simulink model "BT02"  (R2026b)
settings: Solver=ode45  StopTime=cfg.stop_s  MaxStep=cfg.max_step_s  RelTol=1e-10  AbsTol=1e-12
PostLoadFcn:
  | addpath(fileparts(get_param(bdroot,'FileName')));load_case('BT02');
InitFcn:
  | addpath(fileparts(get_param(bdroot,'FileName')));load_case('BT02');
values from neighbouring files (symbols this model uses):
  cfg = jsondecode(fileread(fullfile(root,'fixtures',[id '.json'])))    [load_case.m]
undefined symbols (not defined in the file or in its folder): capacity_Ah, pack_count, solar_gain
settings Model: Creator=markl  LastModifiedBy=markl
settings DataIOCC: SaveOutput=off

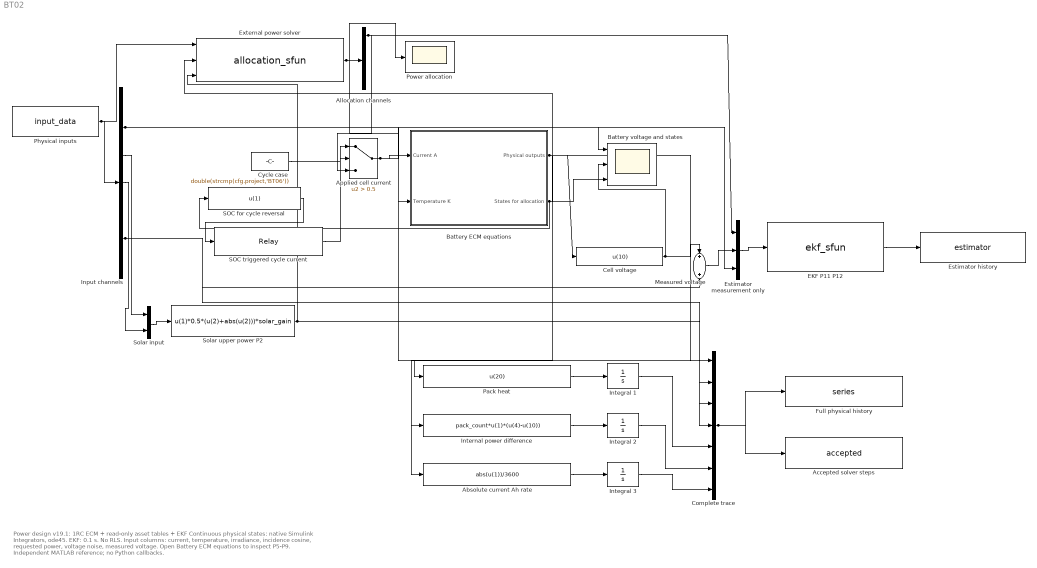
== system BT02 ==
  note: Power design v19.1: 1RC ECM + read-only asset tables + EKF
      | Continuous physical states: native Simulink Integrators, ode45. EKF: 0.1 s. No RLS.
      | Input columns: current, temperature, irradiance, incidence cosine, requested power, voltage noise, measured voltage.
      | Open Battery ECM equations to inspect P5-P9. Independent MATLAB reference; no Python callbacks.
  Absolute current Ah rate : Fcn  Expr=abs(u(1))/3600
  Accepted solver steps : ToWorkspace  VariableName=accepted  SaveFormat=Structure With Time  SampleTime=-1
  Allocation channels : Demux  Outputs=6
  Applied cell current : Switch  Criteria=u2 > Threshold  Threshold=0.5  SaturateOnIntegerOverflow=off  InputSameDT=off
  Battery ECM equations : Subsystem
  Battery voltage and states : Scope  NumInputPorts=3
  Cell voltage : Fcn  Expr=u(10)
  Complete trace : Mux  Inputs=7
  Cycle case : Constant  Value=double(strcmp(cfg.project,'BT06'))
  EKF P11 P12 : M-S-Function  FunctionName=ekf_sfun  Parameters=cfg
  Estimator history : ToWorkspace  VariableName=estimator  SaveFormat=Structure With Time  SampleTime=cfg.dt_s
  Estimator measurement only : Mux  Inputs=3
  External power solver : M-S-Function  FunctionName=allocation_sfun  Parameters=cfg
  Full physical history : ToWorkspace  VariableName=series  SaveFormat=Structure With Time  SampleTime=cfg.dt_s
  Input channels : Demux  Outputs=7
  Integral 1 : Integrator
  Integral 2 : Integrator
  Integral 3 : Integrator
  Internal power difference : Fcn  Expr=pack_count*u(1)*(u(4)-u(10))
  Measured voltage : Sum
  Pack heat : Fcn  Expr=u(20)
  Physical inputs : FromWorkspace  VariableName=input_data  SampleTime=cfg.dt_s  Interpolate=off  OutputAfterFinalValue=Holding final value
  Power allocation : Scope
  SOC for cycle reversal : Fcn  Expr=u(1)
  SOC triggered cycle current : Relay  OnSwitchValue=0.88  OffSwitchValue=0.1  OnOutputValue=0.2  OffOutputValue=-0.2
  Solar input : Mux  Inputs=2
  Solar upper power P2 : Fcn  Expr=u(1)*0.5*(u(2)+abs(u(2)))*solar_gain
  wires:
  Physical inputs/1 -> Input channels/1, External power solver/1
  Input channels/3 -> Solar input/1
  Input channels/4 -> Solar input/2
  Solar input/1 -> Solar upper power P2/1
  Solar upper power P2/1 -> External power solver/3, Complete trace/3
  External power solver/1 -> Allocation channels/1, Complete trace/2, Power allocation/1
  Battery ECM equations/2(States for allocation) -> SOC for cycle reversal/1, External power solver/2, Battery voltage and states/3
  SOC for cycle reversal/1 -> SOC triggered cycle current/1
  SOC triggered cycle current/1 -> Applied cell current/1
  Cycle case/1 -> Applied cell current/2
  Allocation channels/1 -> Applied cell current/3, Estimator measurement only/1
  Applied cell current/1 -> Battery ECM equations/1(Current A), Battery voltage and states/1
  Input channels/2 -> Battery ECM equations/2(Temperature K), Estimator measurement only/3
  Battery ECM equations/1(Physical outputs) -> Cell voltage/1, Pack heat/1, Internal power difference/1, Absolute current Ah rate/1, Complete trace/1
  Cell voltage/1 -> Measured voltage/1, Battery voltage and states/2
  Input channels/6 -> Measured voltage/2, Complete trace/4
  Measured voltage/1 -> Estimator measurement only/2
  Estimator measurement only/1 -> EKF P11 P12/1
  EKF P11 P12/1 -> Estimator history/1
  Pack heat/1 -> Integral 1/1
  Internal power difference/1 -> Integral 2/1
  Absolute current Ah rate/1 -> Integral 3/1
  Integral 1/1 -> Complete trace/5
  Integral 2/1 -> Complete trace/6
  Integral 3/1 -> Complete trace/7
  Complete trace/1 -> Full physical history/1, Accepted solver steps/1

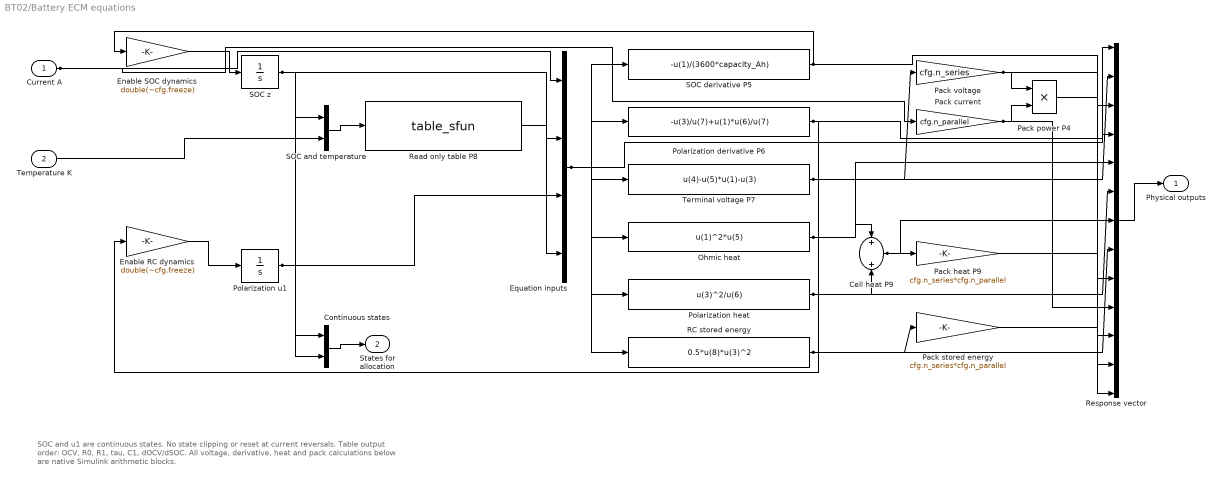
== system BT02/Battery ECM equations ==
  note: SOC and u1 are continuous states. No state clipping or reset at current reversals.
      | Table output order: OCV, R0, R1, tau, C1, dOCV/dSOC.
      | All voltage, derivative, heat and pack calculations below are native Simulink arithmetic blocks.
  Current A : Inport
  Temperature K : Inport  Port=2
  Cell heat P9 : Sum
  Continuous states : Mux  Inputs=2
  Enable RC dynamics : Gain  Gain=double(~cfg.freeze)
  Enable SOC dynamics : Gain  Gain=double(~cfg.freeze)
  Equation inputs : Mux
  Ohmic heat : Fcn  Expr=u(1)^2*u(5)
  Pack current : Gain  Gain=cfg.n_parallel
  Pack heat P9 : Gain  Gain=cfg.n_series*cfg.n_parallel
  Pack power P4 : Product
  Pack stored energy : Gain  Gain=cfg.n_series*cfg.n_parallel
  Pack voltage : Gain  Gain=cfg.n_series
  Polarization derivative P6 : Fcn  Expr=-u(3)/u(7)+u(1)*u(6)/u(7)
  Polarization heat : Fcn  Expr=u(3)^2/u(6)
  Polarization u1 : Integrator  InitialCondition=cfg.initial(2)
  RC stored energy : Fcn  Expr=0.5*u(8)*u(3)^2
  Read only table P8 : M-S-Function  FunctionName=table_sfun  Parameters=cfg
  Response vector : Mux  Inputs=13
  SOC and temperature : Mux  Inputs=2
  SOC derivative P5 : Fcn  Expr=-u(1)/(3600*capacity_Ah)
  SOC z : Integrator  InitialCondition=cfg.initial(1)
  Terminal voltage P7 : Fcn  Expr=u(4)-u(5)*u(1)-u(3)
  Physical outputs : Outport
  States for allocation : Outport  Port=2
  wires:
  SOC z/1 -> SOC and temperature/1, Equation inputs/2, Continuous states/1
  Temperature K/1 -> SOC and temperature/2
  SOC and temperature/1 -> Read only table P8/1
  Current A/1 -> Equation inputs/1, Pack current/1
  Polarization u1/1 -> Equation inputs/3, Continuous states/2
  Read only table P8/1 -> Equation inputs/4
  Equation inputs/1 -> SOC derivative P5/1, Polarization derivative P6/1, Terminal voltage P7/1, Ohmic heat/1, Polarization heat/1, RC stored energy/1, Response vector/1
  SOC derivative P5/1 -> Enable SOC dynamics/1, Response vector/3
  Enable SOC dynamics/1 -> SOC z/1
  Polarization derivative P6/1 -> Enable RC dynamics/1, Response vector/4
  Enable RC dynamics/1 -> Polarization u1/1
  Ohmic heat/1 -> Cell heat P9/1, Response vector/5
  Polarization heat/1 -> Cell heat P9/2, Response vector/6
  Terminal voltage P7/1 -> Pack voltage/1, Response vector/2
  Pack voltage/1 -> Pack power P4/1, Response vector/9
  Pack current/1 -> Pack power P4/2, Response vector/10
  Cell heat P9/1 -> Pack heat P9/1, Response vector/7
  RC stored energy/1 -> Pack stored energy/1, Response vector/8
  Pack power P4/1 -> Response vector/11
  Pack heat P9/1 -> Response vector/12
  Pack stored energy/1 -> Response vector/13
  Response vector/1 -> Physical outputs/1
  Continuous states/1 -> States for allocation/1
